simulink subsystem "s3x3_ULA_RX_from_workspace"  (R2020b)
settings: Solver=VariableStepAuto  StartTime=0.0  StopTime=10.0  RelTol=1e-3
values from neighbouring files (symbols this model uses):
  fs = 1e9    (= 1000000000)    [env_sim_setup.m]
  sv = sv - 0.0001*1i    [env_sim_setup.m]
libraries: simulink x1
settings Model: Creator=jgentile  LastModifiedBy=jgentile

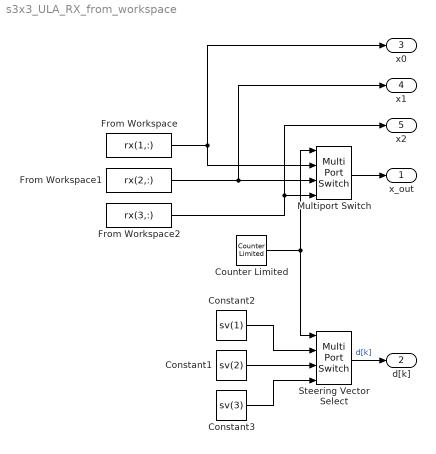
== system s3x3_ULA_RX_from_workspace ==
  Constant1 : Constant  Value=sv(2)
  Constant2 : Constant  Value=sv(1)
  Constant3 : Constant  Value=sv(3)
  Counter Limited : simulink/Sources/Counter Limited  uplimit=2  tsamp=-1
  From Workspace : FromWorkspace  VariableName=rx(1,:)  SampleTime=1/fs
  From Workspace1 : FromWorkspace  VariableName=rx(2,:)  SampleTime=1/fs
  From Workspace2 : FromWorkspace  VariableName=rx(3,:)  SampleTime=1/fs
  Multiport Switch : MultiPortSwitch  DataPortOrder=Zero-based contiguous  zeroidx=on
  Steering Vector Select : MultiPortSwitch  DataPortOrder=Zero-based contiguous  zeroidx=on
  x_out : Outport
  d[k] : Outport  Port=2
      settings: SignalType=complex
  x0 : Outport  Port=3
  x1 : Outport  Port=4
  x2 : Outport  Port=5
  wires:
  Constant1/1 -> Steering Vector Select/3
  Constant3/1 -> Steering Vector Select/4
  Multiport Switch/1 -> x_out/1
  Steering Vector Select/1 -> d[k]/1  "d[k]"
  Counter Limited/1 -> Multiport Switch/1, Steering Vector Select/1
  Constant2/1 -> Steering Vector Select/2
  From Workspace2/1 -> Multiport Switch/4, x2/1
  From Workspace1/1 -> x1/1, Multiport Switch/3
  From Workspace/1 -> Multiport Switch/2, x0/1
